simulink model "pendulum_model"  (R2025b)
settings: Solver=FixedStepAuto  StartTime=0.0  StopTime=50  FixedStep=0.01  RelTol=1e-3
values from neighbouring files (symbols this model uses):
  G_fii = -0.008456    [run_simulink_model.m]    (also in tune_model.m)
  G_t = 4.097306    [run_simulink_model.m]    (also in tune_model.m)
  G_tp = -0.152144    [run_simulink_model.m]    (also in tune_model.m)
  Gfi = -1.045953    [run_simulink_model.m]    (also in tune_model.m)
  Gu = 457.443480    (= 457.44348)    [run_simulink_model.m]    (also in tune_model.m)
  useSignForFrict = 1    [run_simulink_model.m]    (also in tune_model.m = 0)
  withMotor = 1    [run_simulink_model.m]    (also in tune_model.m)
  x0_state = [pendVel(1), pendPosZU(1)]    [run_simulink_model.m]
settings Model: Creator=igorsiata  LastModifiedBy=igorsiata

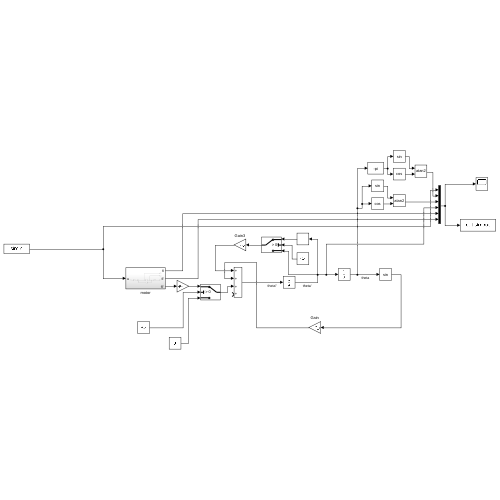
[thumbnail: Simulink's stored preview of the top-level diagram]
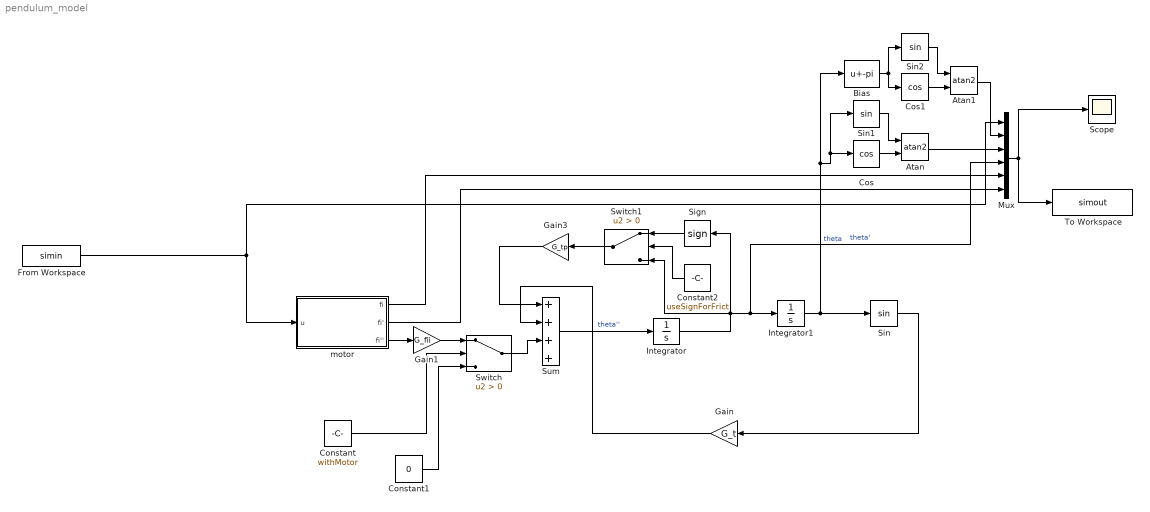
== system pendulum_model ==
  Atan : Trigonometry  Operator=atan2
  Atan1 : Trigonometry  Operator=atan2
  Bias : Bias  Bias=-pi  SaturateOnIntegerOverflow=off
  Constant : Constant  Value=withMotor
  Constant1 : Constant  Value=0
  Constant2 : Constant  Value=useSignForFrict
  Cos : Trigonometry  Operator=cos
  Cos1 : Trigonometry  Operator=cos
  From Workspace : FromWorkspace  VariableName=simin
  Gain : Gain  Gain=G_t
  Gain1 : Gain  Gain=G_fii
  Gain3 : Gain  Gain=G_tp
  Integrator : Integrator  InitialCondition=x0_state(1)
  Integrator1 : Integrator  InitialCondition=x0_state(2)
  Mux : Mux  Inputs=6
  Scope : Scope
      settings: ActiveDisplayYMinimum=-41592.647928357357  ActiveDisplayYMaximum=69394.182930693918
  Sign : Signum
  Sin : Trigonometry
  Sin1 : Trigonometry
  Sin2 : Trigonometry
  Sum : Sum  Inputs=++++
  Switch : Switch  Criteria=u2 > Threshold  SaturateOnIntegerOverflow=off  InputSameDT=off
  Switch1 : Switch  Criteria=u2 > Threshold  SaturateOnIntegerOverflow=off  InputSameDT=off
  To Workspace : ToWorkspace  VariableName=simout  SaveFormat=Timeseries  SampleTime=-1
  motor : Subsystem
  wires:
  Integrator/1 -> Switch1/3, Sign/1, Mux/4, Integrator1/1  "theta'"
  Mux/1 -> To Workspace/1, Scope/1
  Integrator1/1 -> Bias/1, Sin1/1, Cos/1, Sin/1  "theta"
  Sum/1 -> Integrator/1  "theta''"
  Gain3/1 -> Sum/1
  Gain/1 -> Sum/2
  Sin/1 -> Gain/1
  From Workspace/1 -> motor/1(u), Mux/1
  motor/3(fi'') -> Gain1/1
  Sign/1 -> Switch1/1
  motor/1(fi) -> Mux/5
  motor/2(fi') -> Mux/6
  Gain1/1 -> Switch/1
  Switch/1 -> Sum/3
  Constant/1 -> Switch/2
  Constant1/1 -> Switch/3
  Switch1/1 -> Gain3/1
  Constant2/1 -> Switch1/2
  Sin1/1 -> Atan/1
  Cos/1 -> Atan/2
  Atan/1 -> Mux/3
  Sin2/1 -> Atan1/1
  Cos1/1 -> Atan1/2
  Bias/1 -> Cos1/1, Sin2/1
  Atan1/1 -> Mux/2

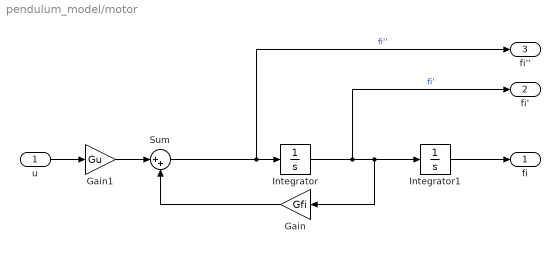
== system pendulum_model/motor ==
  u : Inport
  Gain : Gain  Gain=Gfi
  Gain1 : Gain  Gain=Gu
  Integrator : Integrator
  Integrator1 : Integrator
  Sum : Sum  Inputs=|++
  fi : Outport
  fi' : Outport  Port=2
  fi'' : Outport  Port=3
  wires:
  Gain/1 -> Sum/2
  Gain1/1 -> Sum/1
  u/1 -> Gain1/1
  Integrator/1 -> fi'/1, Gain/1, Integrator1/1  "fi'"
  Sum/1 -> fi''/1, Integrator/1  "fi''"
  Integrator1/1 -> fi/1
